simulink model "final_sim_v3_2023a"  (R2023b)
settings: Solver=VariableStepAuto  StartTime=0.0  StopTime=20  RelTol=1e-3
libraries: simulink_extras x2, simulink x2
settings Model: Creator=user  LastModifiedBy=ian20030201
settings RTWCC: GPUComputeCapability=5.0

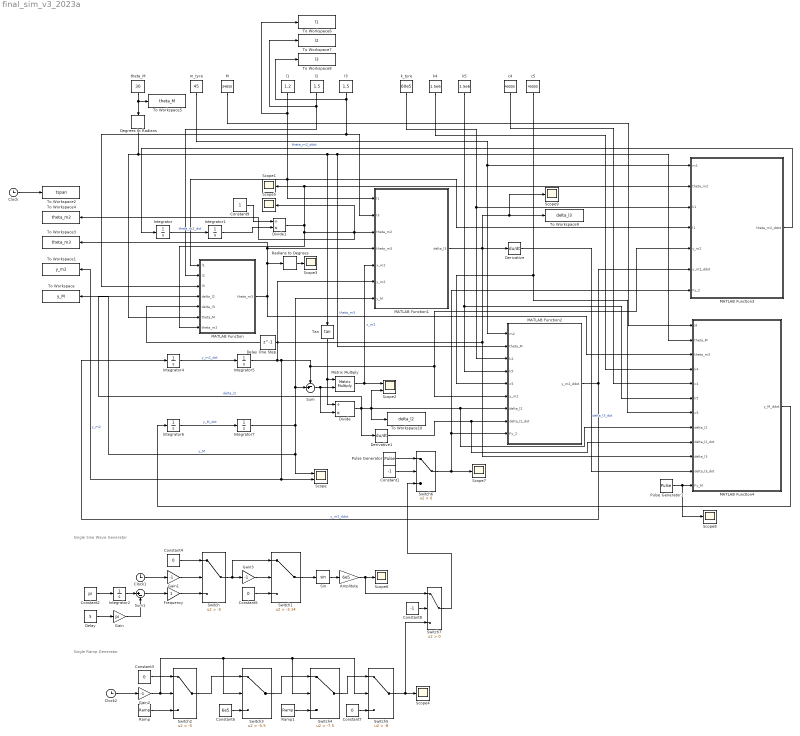
== system final_sim_v3_2023a ==
  note: Single Ramp Generator
  note: Single Sine Wave Generator
  Amplitute : Gain  Gain=6e5
  Clock : Clock
  Clock1 : Clock
  Clock2 : Clock
  Constant1 : Constant  Value=-1
  Constant2 : Constant  Value=pi
  Constant{3..5,7} (4 alike) : Constant  Value=0
  Constant6 : Constant  Value=6e5
  Constant8 : Constant  Value=-1
  Constant9 : Constant
  Degrees to Radians : simulink_extras/Transformations/Degrees to Radians
  Delay : Constant  Value=5
  Delay One Step : Delay  DelayLength=1
  Derivative : Derivative
  Derivative1 : Derivative
  Divide : Product  Inputs=/*
  Divide1 : Product  Inputs=/*
  Frequency : Gain
  Gain : Gain  Gain=pi
  Gain1 : Gain  Gain=-1
  Gain2 : Gain  Gain=-1
  Gain3 : Gain  Gain=-1
  Integrator{,1..2,4..7} (7 alike) : Integrator
  M : Constant  Value=34850
  MATLAB Function : MATLAB Function  TreatAsAtomicUnit=on
  MATLAB Function1 : MATLAB Function  TreatAsAtomicUnit=on
  MATLAB Function2 : MATLAB Function  TreatAsAtomicUnit=on
  MATLAB Function3 : MATLAB Function  TreatAsAtomicUnit=on
  MATLAB Function4 : MATLAB Function  TreatAsAtomicUnit=on
  Matrix Multiply : Product  Multiplication=Matrix(*)
  Pulse Generator : DiscretePulseGenerator  PulseType=Time based  Amplitude=6e5  Period=20  PulseWidth=5  PhaseDelay=5
  Pulse Generator1 : DiscretePulseGenerator  PulseType=Time based  Amplitude=-34850*9.81  Period=100  PulseWidth=90  PhaseDelay=8
  Radians to Degrees : simulink_extras/Transformations/Radians to Degrees
  Ramp : simulink/Sources/Ramp  slope=6e5/0.5  start=5  InitialOutput=0
  Ramp1 : simulink/Sources/Ramp  slope=-6e5/0.5  start=7.5  InitialOutput=6e5
  Scope : Scope  NumInputPorts=2
  Scope{1,3..9} (8 alike) : Scope
  Scope2 : Scope  NumInputPorts=2
  Sin : Trigonometry
  Sum : Sum  Inputs=-+|
  Sum1 : Sum  Inputs=|+-
  Switch : Switch  Criteria=u2 > Threshold  Threshold=-5  SaturateOnIntegerOverflow=off  InputSameDT=off
  Switch1 : Switch  Criteria=u2 > Threshold  Threshold=-3.14  SaturateOnIntegerOverflow=off  InputSameDT=off
  Switch2 : Switch  Criteria=u2 > Threshold  Threshold=-5  SaturateOnIntegerOverflow=off  InputSameDT=off
  Switch3 : Switch  Criteria=u2 > Threshold  Threshold=-5.5  SaturateOnIntegerOverflow=off  InputSameDT=off
  Switch4 : Switch  Criteria=u2 > Threshold  Threshold=-7.5  SaturateOnIntegerOverflow=off  InputSameDT=off
  Switch5 : Switch  Criteria=u2 > Threshold  Threshold=-8  SaturateOnIntegerOverflow=off  InputSameDT=off
  Switch6 : Switch  Criteria=u2 > Threshold  SaturateOnIntegerOverflow=off  InputSameDT=off
  Switch7 : Switch  Criteria=u2 > Threshold  SaturateOnIntegerOverflow=off  InputSameDT=off
  Tan : Trigonometry  Operator=tan
  To Workspace : ToWorkspace  VariableName=y_M  SampleTime=0.05
      settings: Save2DSignal=2-D array (concatenate along first dimension)
  To Workspace1 : ToWorkspace  VariableName=y_m2  SampleTime=0.05
      settings: Save2DSignal=2-D array (concatenate along first dimension)
  To Workspace10 : ToWorkspace  VariableName=delta_l2  SampleTime=0.05
  To Workspace2 : ToWorkspace  VariableName=tspan  SampleTime=0.05
  To Workspace3 : ToWorkspace  VariableName=theta_m3  SampleTime=0.05
      settings: Save2DSignal=2-D array (concatenate along first dimension)
  To Workspace4 : ToWorkspace  VariableName=theta_m2  SampleTime=0.05
      settings: Save2DSignal=2-D array (concatenate along first dimension)
  To Workspace5 : ToWorkspace  VariableName=theta_M  SampleTime=-1
  To Workspace6 : ToWorkspace  VariableName=l1  SampleTime=-1
  To Workspace7 : ToWorkspace  VariableName=l2  SampleTime=-1
  To Workspace8 : ToWorkspace  VariableName=l3  SampleTime=-1
  To Workspace9 : ToWorkspace  VariableName=delta_l3  SampleTime=0.05
      settings: Save2DSignal=2-D array (concatenate along first dimension)
  c4 : Constant  Value=40000
  c5 : Constant  Value=40000
  k4 : Constant  Value=1.5e6
  k5 : Constant  Value=1.5e6
  k_tyre : Constant  Value=60e5
  l1 : Constant  Value=1.2
  l2 : Constant  Value=1.5
  l3 : Constant  Value=1.5
  m_tyre : Constant  Value=45
  theta_M : Constant  Value=30
  wires:
  MATLAB Function3/1(theta_m2_ddot) -> Integrator/1  "theta_m2_ddot"
  Integrator/1 -> Integrator1/1  "theta_m2_dot"
  MATLAB Function2/1(y_m2_ddot) -> MATLAB Function3/6(y_m2_ddot), Integrator4/1  "y_m2_ddot"
  Integrator4/1 -> Integrator5/1  "y_m2_dot"
  Integrator6/1 -> Integrator7/1  "y_M_dot"
  Divide1/1 -> MATLAB Function/7(theta_m2), Scope5/1, To Workspace4/1, MATLAB Function1/3(theta_m2), Scope1/1, MATLAB Function3/2(theta_m2)
  MATLAB Function/1(theta_m3) -> MATLAB Function4/3(theta_m3), MATLAB Function1/4(theta_m3), To Workspace3/1, Radians to Degrees/1  "theta_m3"
  Integrator5/1 -> Scope/2, To Workspace1/1, MATLAB Function2/6(y_m2), MATLAB Function3/5(y_m2), Sum/1, MATLAB Function1/6(y_m2)  "y_m2"
  Integrator7/1 -> To Workspace/1, Scope/1, Sum/2, MATLAB Function1/7(y_M)  "y_M"
  l1/1 -> To Workspace6/1, MATLAB Function/1(l1), MATLAB Function3/4(l1), MATLAB Function1/1(l1)
  l3/1 -> MATLAB Function/3(l3), MATLAB Function1/2(l3), To Workspace8/1
  Tan/1 -> Divide/1, Matrix Multiply/1
  Sum/1 -> Divide/2, Matrix Multiply/2
  theta_M/1 -> Degrees to Radians/1, To Workspace5/1
  Matrix Multiply/1 -> MATLAB Function1/5(x_m2), Scope2/1  "x_m2"
  Divide/1 -> MATLAB Function/4(delta_l2), To Workspace10/1, Scope2/2, MATLAB Function4/8(delta_l2), MATLAB Function2/7(delta_l2), Derivative1/1  "delta_l2"
  MATLAB Function1/1(delta_l3) -> Scope9/1, To Workspace9/1, Derivative/1, MATLAB Function4/10(delta_l3), Delay One Step/1
  Derivative/1 -> MATLAB Function4/11(delta_l3_dot)  "delta_l3_dot"
  Derivative1/1 -> MATLAB Function4/9(delta_l2_dot), MATLAB Function2/8(delta_l2_dot)
  Amplitute/1 -> Switch7/1, Scope6/1
  k5/1 -> MATLAB Function4/6(k5), MATLAB Function2/4(k5)
  c5/1 -> MATLAB Function4/7(c5), MATLAB Function2/5(c5)
  k_tyre/1 -> MATLAB Function2/3(k2), MATLAB Function3/3(k1)
  m_tyre/1 -> MATLAB Function2/1(m2), MATLAB Function3/1(m1)
  Pulse Generator1/1 -> Scope8/1, MATLAB Function4/12(Fy_M)
  MATLAB Function4/1(y_M_ddot) -> Integrator6/1
  M/1 -> MATLAB Function4/1(M)
  k4/1 -> MATLAB Function4/4(k4)
  c4/1 -> MATLAB Function4/5(c4)
  l2/1 -> MATLAB Function/2(l2), To Workspace7/1
  Delay One Step/1 -> MATLAB Function/5(delta_l3)
  Degrees to Radians/1 -> MATLAB Function/6(theta_M), Tan/1, MATLAB Function4/2(theta_M), MATLAB Function2/2(theta_M)
  Radians to Degrees/1 -> Scope3/1
  Clock/1 -> To Workspace2/1
  Constant2/1 -> Integrator2/1
  Integrator2/1 -> Sum1/1
  Delay/1 -> Gain/1
  Gain/1 -> Sum1/2
  Constant4/1 -> Switch/1
  Clock1/1 -> Gain1/1
  Gain1/1 -> Switch/2
  Sum1/1 -> Frequency/1
  Frequency/1 -> Switch/3
  Switch/1 -> Switch1/1, Gain3/1
  Gain3/1 -> Switch1/2
  Switch1/1 -> Sin/1
  Constant5/1 -> Switch1/3
  Sin/1 -> Amplitute/1
  Gain2/1 -> Switch5/2, Switch4/2, Switch3/2, Switch2/2
  Clock2/1 -> Gain2/1
  Constant3/1 -> Switch2/1
  Ramp/1 -> Switch2/3
  Switch2/1 -> Switch3/1
  Constant6/1 -> Switch3/3
  Switch3/1 -> Switch4/1
  Switch4/1 -> Switch5/1
  Switch5/1 -> Switch7/3, Scope4/1
  Constant7/1 -> Switch5/3
  Ramp1/1 -> Switch4/3
  Switch6/1 -> MATLAB Function3/7(Fy_2), MATLAB Function2/9(Fy_2), Scope7/1
  Pulse Generator/1 -> Switch6/1
  Constant1/1 -> Switch6/2
  Switch7/1 -> Switch6/3
  Constant8/1 -> Switch7/2
  Constant9/1 -> Divide1/1
  Integrator1/1 -> Divide1/2

== matlab function final_sim_v3_2023a/MATLAB Function1 ==
  data: delta_l3 output; l1 input; l3 input; theta_m2 input; theta_m3 input; x_m2 input; y_m2 input; y_M input
function delta_l3 = fcn(l1, l3, theta_m2, theta_m3, x_m2, y_m2, y_M)

l3_t = sqrt((l3*sin(theta_m3)-x_m2)^2 + (l3*cos(theta_m3)-(y_m2-l1*theta_m2)+y_M)^2);
delta_l3 = l3_t - l3;

== matlab function final_sim_v3_2023a/MATLAB Function2 ==
  data: m2 input; theta_M input; k2 input; k5 input; c5 input; y_m2 input; delta_l2 input; delta_l2_dot input; Fy_2 input; y_m2_ddot output
function y_m2_ddot = fcn(m2, theta_M, k2, k5, c5, y_m2, delta_l2, delta_l2_dot, Fy_2)

g = 0;
y_m2_ddot = (Fy_2 + (k5*delta_l2 + c5*delta_l2_dot)*cos(theta_M) - m2*g -k2*y_m2)/m2;

== matlab function final_sim_v3_2023a/MATLAB Function3 ==
  data: m1 input; theta_m2 input; k1 input; l1 input; y_m2 input; y_m2_ddot input; theta_m2_ddot output; Fy_2 input
function theta_m2_ddot = fcn(m1, theta_m2, k1, l1, y_m2, y_m2_ddot, Fy_2)

g = 0;
theta_m2_ddot = (((-m1*g - k1*(y_m2 + l1*theta_m2) + Fy_2)/m1) - y_m2_ddot)/l1;

== matlab function final_sim_v3_2023a/MATLAB Function4 ==
  data: M input; theta_M input; theta_m3 input; k4 input; c4 input; k5 input; y_M_ddot output; c5 input; delta_l2 input; delta_l2_dot input; delta_l3 input; delta_l3_dot input; Fy_M input
function y_M_ddot = fcn(M, theta_M, theta_m3, k4, c4, k5, c5, delta_l2, delta_l2_dot, delta_l3, delta_l3_dot, Fy_M)

g = 0;
y_M_ddot = (Fy_M - (k4*delta_l3 + c4*delta_l3_dot)*cos(theta_m3) - M*g - (k5*delta_l2 + c5*delta_l2_dot)*cos(theta_M))/M;

== matlab function final_sim_v3_2023a/MATLAB Function ==
  data: l1 input; theta_m3 output; l2 input; l3 input; delta_l2 input; delta_l3 input; theta_M input; theta_m2 input
function theta_m3 = fcn(l1, l2, l3, delta_l2, delta_l3, theta_M, theta_m2)

slope = (l3+delta_l3);
side_1 = ((l2+delta_l2)*cos(theta_M)+l1*sin(theta_m2));
side_2 = sqrt(abs(slope^2 - side_1^2));
theta_m3 = atan(side_2/side_1);
